simulink model "Quadcopter_sim1NEW"  (R2021a)
settings: Solver=VariableStepAuto  StartTime=0.0  StopTime=t_stop  RelTol=1e-3
values from neighbouring files (symbols this model uses):
  b = 0.001    [Exercise2.m]    (also in Exercise2_3.m)
  Dx = 0.01    [Exercise2.m]    (also in Exercise2_3.m)
  Dy = 0.01    [Exercise2.m]    (also in Exercise2_3.m)
  Dz = 0.01    [Exercise2.m]    (also in Exercise2_3.m)
  g = 9.81    [Exercise2.m]    (also in Exercise2_3.m)
  Ixx = 3e-06    [Exercise2.m]    (also in Exercise2_3.m)
  Iyy = 3e-06    [Exercise2.m]    (also in Exercise2_3.m)
  Izz = 1e-05    [Exercise2.m]    (also in Exercise2_3.m)
  k = 0.01    [Exercise2.m]    (also in Exercise2_3.m)
  L = 0.225    [Exercise2.m]    (also in Exercise2_3.m)
  m = 0.5    [Exercise2.m]    (also in Exercise2_3.m)
  phiSP = phiDegree*pi/180    (= 0)    [Exercise2.m]
  psiSP = psiDegree*pi/180    (= 0)    [Exercise2.m]
  thetaSP = thetaDegree*pi/180    (= 0)    [Exercise2.m]
  zSP = 10    [Exercise2.m]
libraries: pid_lib x4, vrlib x1
settings Model: Creator=emilm  LastModifiedBy=emilm

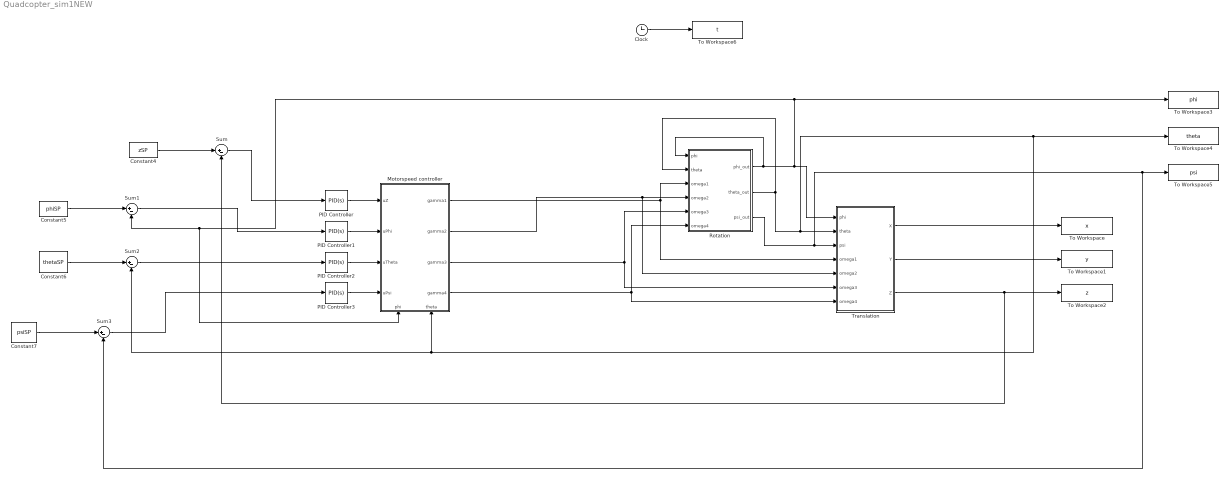
== system Quadcopter_sim1NEW ==
  Clock : Clock
  Constant4 : Constant  Value=zSP
  Constant5 : Constant  Value=phiSP
  Constant6 : Constant  Value=thetaSP
  Constant7 : Constant  Value=psiSP
  Motorspeed controller : Subsystem
      settings: PortSchema="{\"entries\":[{\"content\":{\"sides\":[{\"content\":{\"connectorIds\":[\"In1\",\"In2\",\"In3\",\"In4\"]},\"type\":\"ConnectorPlacement.EquallySpacedRectSide\",\"uuid\":\"02bb1367-ab6e-4bd8-8433-2a069659d175\"},{\"content\":{\"connectorIds\":[\"Out1\",\"Out2\",\"Out3\",\"Out4\"],\"side\":\"RIGHT\"},\"type\":\"ConnectorPlacement.EquallySpacedRectSide\",\"uuid\":\"a63fe295-d221-4681-8f7c-a69bc5358675\"},{\"content\":{\"connectorIds\":[],\"side\":\"TOP\"},\"type\":\"ConnectorPlacement.EquallySpacedRectSide\",\"uuid\":\"253ed6a3-3e04-4ad6-995f-50a6275cee5f\"},{\"content\":{\"connectorIds\":[\"In5\",\"In6\"],\"side\":\"BOTTOM\"},\"type\":\"ConnectorPlacement.EquallySpacedRectSide\",\"uuid\":\"f5e775ff-abe8-4d7a-a704-f626c46163f8\"}]},\"type\":\"ConnectorPlacement.EquallySpacedConnector\",\"uuid\":\"7d3e2221-d52d-4562-8edc-19cce75af537\"}],\"packageUris\":[\"http://schema.mathworks.com/mf0/Connector/R2020b\"],\"version\":\"1.0\"}"
  PID Controller : pid_lib/PID Controller  Controller=PID  Form=Parallel  TimeDomain=Continuous-time  UseExternalTs=off  SampleTime=-1  IntegratorMethod=Forward Euler  FilterMethod=Forward Euler  ControllerParametersSource=internal  P=4.3  I=4.5  D=2  UseFilter=on  N=100  TunerSelectOption=Transfer Function Based (PID Tuner App)  InitialConditionSource=internal  InitialConditionForIntegrator=0  InitialConditionForFilter=0  DifferentiatorICPrevScaledInput=0  ExternalReset=none  TrackingMode=off  Kt=1  LimitOutput=off  SatLimitsSource=internal  UpperSaturationLimit=inf  LowerSaturationLimit=-inf  LinearizeAsGain=on  AntiWindupMode=none  Kb=1  POutMin=[]  POutMax=[]  IOutMin=[]  IOutMax=[]  DOutMin=[]  DOutMax=[]  NOutMin=[]  NOutMax=[]  SumOutMin=[]  SumOutMax=[]  SaturationOutMin=[]  SaturationOutMax=[]  PParamMin=[]  PParamMax=[]  IParamMin=[]  IParamMax=[]  DParamMin=[]  DParamMax=[]  NParamMin=[]  NParamMax=[]  KbParamMin=[]  KbParamMax=[]  KtParamMin=[]  KtParamMax=[]  KbOutMin=[]  KbOutMax=[]  KtOutMin=[]  KtOutMax=[]  IntegratorOutMin=[]  IntegratorOutMax=[]  FilterOutMin=[]  FilterOutMax=[]  SumI1OutMin=[]  SumI1OutMax=[]  SumI2OutMin=[]  SumI2OutMax=[]  SumI3OutMin=[]  SumI3OutMax=[]  SumI4OutMin=[]  SumI4OutMax=[]  SumDOutMin=[]  SumDOutMax=[]  DifferentiatorOutMin=[]  DifferentiatorOutMax=[]  FilterDiffOutCoefMin=[]  FilterDiffOutCoefMax=[]  ReciprocalOutMin=[]  ReciprocalOutMax=[]  SumDenOutMin=[]  SumDenOutMax=[]  SumNumOutMin=[]  SumNumOutMax=[]  DivideOutMin=[]  DivideOutMax=[]  UdiffTsProdOutMin=[]  UdiffTsProdOutMax=[]  NTsProdOutMin=[]  NTsProdOutMax=[]  UintegralTsProdOutMin=[]  UintegralTsProdOutMax=[]  UngainTsProdOutMin=[]  UngainTsProdOutMax=[]  IntegratorContinuousStateAttributes=''  IntegratorStateMustResolveToSignalObject=off  IntegratorRTWStateStorageClass=Auto  FilterContinuousStateAttributes=''  FilterStateMustResolveToSignalObject=off  FilterRTWStateStorageClass=Auto  ParallelPVariant=InternalParameters  IdealPVariant=Disabled  IVariant=InternalParameters  DVariant=InternalParameters  IntegratorVariant=Continuous  SatVariant=Disabled  AWVariant=Passthrough  PCopyVariant=Disabled  TRVariant=Disabled  FdbkBlocksVariant=Forward  IdealPFdbkVariant=Disabled  SatFdbkVariant=Disabled  DerivativeFilterVariant=ContFilter  NVariant=InternalParameters  NCopyVariant=Disabled  FilterICVariant=InternalICsFilter  IntegratorICVariant=InternalICs  ExternalResetVariant=Disabled  TRSumVariant=Passthrough  SumFdbkVariant=Disabled  SumVariant=Sum_PID  TsampFilterVariant=InternalTs  TsampNgainVariant=Passthrough  TsampIntegralVariant=Passthrough  ExternalSaturationOutDataTypeStr=Inherit: Same as second input
  PID Controller1 : pid_lib/PID Controller  Controller=PID  Form=Parallel  TimeDomain=Continuous-time  UseExternalTs=off  SampleTime=-1  IntegratorMethod=Forward Euler  FilterMethod=Forward Euler  ControllerParametersSource=internal  P=0.006  I=0.000009  D=0.013  UseFilter=on  N=100  TunerSelectOption=Transfer Function Based (PID Tuner App)  InitialConditionSource=internal  InitialConditionForIntegrator=0  InitialConditionForFilter=0  DifferentiatorICPrevScaledInput=0  ExternalReset=none  TrackingMode=off  Kt=1  LimitOutput=off  SatLimitsSource=internal  UpperSaturationLimit=inf  LowerSaturationLimit=-inf  LinearizeAsGain=on  AntiWindupMode=none  Kb=1  POutMin=[]  POutMax=[]  IOutMin=[]  IOutMax=[]  DOutMin=[]  DOutMax=[]  NOutMin=[]  NOutMax=[]  SumOutMin=[]  SumOutMax=[]  SaturationOutMin=[]  SaturationOutMax=[]  PParamMin=[]  PParamMax=[]  IParamMin=[]  IParamMax=[]  DParamMin=[]  DParamMax=[]  NParamMin=[]  NParamMax=[]  KbParamMin=[]  KbParamMax=[]  KtParamMin=[]  KtParamMax=[]  KbOutMin=[]  KbOutMax=[]  KtOutMin=[]  KtOutMax=[]  IntegratorOutMin=[]  IntegratorOutMax=[]  FilterOutMin=[]  FilterOutMax=[]  SumI1OutMin=[]  SumI1OutMax=[]  SumI2OutMin=[]  SumI2OutMax=[]  SumI3OutMin=[]  SumI3OutMax=[]  SumI4OutMin=[]  SumI4OutMax=[]  SumDOutMin=[]  SumDOutMax=[]  DifferentiatorOutMin=[]  DifferentiatorOutMax=[]  FilterDiffOutCoefMin=[]  FilterDiffOutCoefMax=[]  ReciprocalOutMin=[]  ReciprocalOutMax=[]  SumDenOutMin=[]  SumDenOutMax=[]  SumNumOutMin=[]  SumNumOutMax=[]  DivideOutMin=[]  DivideOutMax=[]  UdiffTsProdOutMin=[]  UdiffTsProdOutMax=[]  NTsProdOutMin=[]  NTsProdOutMax=[]  UintegralTsProdOutMin=[]  UintegralTsProdOutMax=[]  UngainTsProdOutMin=[]  UngainTsProdOutMax=[]  IntegratorContinuousStateAttributes=''  IntegratorStateMustResolveToSignalObject=off  IntegratorRTWStateStorageClass=Auto  FilterContinuousStateAttributes=''  FilterStateMustResolveToSignalObject=off  FilterRTWStateStorageClass=Auto  ParallelPVariant=InternalParameters  IdealPVariant=Disabled  IVariant=InternalParameters  DVariant=InternalParameters  IntegratorVariant=Continuous  SatVariant=Disabled  AWVariant=Passthrough  PCopyVariant=Disabled  TRVariant=Disabled  FdbkBlocksVariant=Forward  IdealPFdbkVariant=Disabled  SatFdbkVariant=Disabled  DerivativeFilterVariant=ContFilter  NVariant=InternalParameters  NCopyVariant=Disabled  FilterICVariant=InternalICsFilter  IntegratorICVariant=InternalICs  ExternalResetVariant=Disabled  TRSumVariant=Passthrough  SumFdbkVariant=Disabled  SumVariant=Sum_PID  TsampFilterVariant=InternalTs  TsampNgainVariant=Passthrough  TsampIntegralVariant=Passthrough  ExternalSaturationOutDataTypeStr=Inherit: Same as second input
  PID Controller2 : pid_lib/PID Controller  Controller=PID  Form=Parallel  TimeDomain=Continuous-time  UseExternalTs=off  SampleTime=-1  IntegratorMethod=Forward Euler  FilterMethod=Forward Euler  ControllerParametersSource=internal  P=0.006  I=0.000009  D=0.013  UseFilter=on  N=100  TunerSelectOption=Transfer Function Based (PID Tuner App)  InitialConditionSource=internal  InitialConditionForIntegrator=0  InitialConditionForFilter=0  DifferentiatorICPrevScaledInput=0  ExternalReset=none  TrackingMode=off  Kt=1  LimitOutput=off  SatLimitsSource=internal  UpperSaturationLimit=inf  LowerSaturationLimit=-inf  LinearizeAsGain=on  AntiWindupMode=none  Kb=1  POutMin=[]  POutMax=[]  IOutMin=[]  IOutMax=[]  DOutMin=[]  DOutMax=[]  NOutMin=[]  NOutMax=[]  SumOutMin=[]  SumOutMax=[]  SaturationOutMin=[]  SaturationOutMax=[]  PParamMin=[]  PParamMax=[]  IParamMin=[]  IParamMax=[]  DParamMin=[]  DParamMax=[]  NParamMin=[]  NParamMax=[]  KbParamMin=[]  KbParamMax=[]  KtParamMin=[]  KtParamMax=[]  KbOutMin=[]  KbOutMax=[]  KtOutMin=[]  KtOutMax=[]  IntegratorOutMin=[]  IntegratorOutMax=[]  FilterOutMin=[]  FilterOutMax=[]  SumI1OutMin=[]  SumI1OutMax=[]  SumI2OutMin=[]  SumI2OutMax=[]  SumI3OutMin=[]  SumI3OutMax=[]  SumI4OutMin=[]  SumI4OutMax=[]  SumDOutMin=[]  SumDOutMax=[]  DifferentiatorOutMin=[]  DifferentiatorOutMax=[]  FilterDiffOutCoefMin=[]  FilterDiffOutCoefMax=[]  ReciprocalOutMin=[]  ReciprocalOutMax=[]  SumDenOutMin=[]  SumDenOutMax=[]  SumNumOutMin=[]  SumNumOutMax=[]  DivideOutMin=[]  DivideOutMax=[]  UdiffTsProdOutMin=[]  UdiffTsProdOutMax=[]  NTsProdOutMin=[]  NTsProdOutMax=[]  UintegralTsProdOutMin=[]  UintegralTsProdOutMax=[]  UngainTsProdOutMin=[]  UngainTsProdOutMax=[]  IntegratorContinuousStateAttributes=''  IntegratorStateMustResolveToSignalObject=off  IntegratorRTWStateStorageClass=Auto  FilterContinuousStateAttributes=''  FilterStateMustResolveToSignalObject=off  FilterRTWStateStorageClass=Auto  ParallelPVariant=InternalParameters  IdealPVariant=Disabled  IVariant=InternalParameters  DVariant=InternalParameters  IntegratorVariant=Continuous  SatVariant=Disabled  AWVariant=Passthrough  PCopyVariant=Disabled  TRVariant=Disabled  FdbkBlocksVariant=Forward  IdealPFdbkVariant=Disabled  SatFdbkVariant=Disabled  DerivativeFilterVariant=ContFilter  NVariant=InternalParameters  NCopyVariant=Disabled  FilterICVariant=InternalICsFilter  IntegratorICVariant=InternalICs  ExternalResetVariant=Disabled  TRSumVariant=Passthrough  SumFdbkVariant=Disabled  SumVariant=Sum_PID  TsampFilterVariant=InternalTs  TsampNgainVariant=Passthrough  TsampIntegralVariant=Passthrough  ExternalSaturationOutDataTypeStr=Inherit: Same as second input
  PID Controller3 : pid_lib/PID Controller  Controller=PID  Form=Parallel  TimeDomain=Continuous-time  UseExternalTs=off  SampleTime=-1  IntegratorMethod=Forward Euler  FilterMethod=Forward Euler  ControllerParametersSource=internal  P=0.01  I=0.0002  D=0.03  UseFilter=on  N=100  TunerSelectOption=Transfer Function Based (PID Tuner App)  InitialConditionSource=internal  InitialConditionForIntegrator=0  InitialConditionForFilter=0  DifferentiatorICPrevScaledInput=0  ExternalReset=none  TrackingMode=off  Kt=1  LimitOutput=off  SatLimitsSource=internal  UpperSaturationLimit=inf  LowerSaturationLimit=-inf  LinearizeAsGain=on  AntiWindupMode=none  Kb=1  POutMin=[]  POutMax=[]  IOutMin=[]  IOutMax=[]  DOutMin=[]  DOutMax=[]  NOutMin=[]  NOutMax=[]  SumOutMin=[]  SumOutMax=[]  SaturationOutMin=[]  SaturationOutMax=[]  PParamMin=[]  PParamMax=[]  IParamMin=[]  IParamMax=[]  DParamMin=[]  DParamMax=[]  NParamMin=[]  NParamMax=[]  KbParamMin=[]  KbParamMax=[]  KtParamMin=[]  KtParamMax=[]  KbOutMin=[]  KbOutMax=[]  KtOutMin=[]  KtOutMax=[]  IntegratorOutMin=[]  IntegratorOutMax=[]  FilterOutMin=[]  FilterOutMax=[]  SumI1OutMin=[]  SumI1OutMax=[]  SumI2OutMin=[]  SumI2OutMax=[]  SumI3OutMin=[]  SumI3OutMax=[]  SumI4OutMin=[]  SumI4OutMax=[]  SumDOutMin=[]  SumDOutMax=[]  DifferentiatorOutMin=[]  DifferentiatorOutMax=[]  FilterDiffOutCoefMin=[]  FilterDiffOutCoefMax=[]  ReciprocalOutMin=[]  ReciprocalOutMax=[]  SumDenOutMin=[]  SumDenOutMax=[]  SumNumOutMin=[]  SumNumOutMax=[]  DivideOutMin=[]  DivideOutMax=[]  UdiffTsProdOutMin=[]  UdiffTsProdOutMax=[]  NTsProdOutMin=[]  NTsProdOutMax=[]  UintegralTsProdOutMin=[]  UintegralTsProdOutMax=[]  UngainTsProdOutMin=[]  UngainTsProdOutMax=[]  IntegratorContinuousStateAttributes=''  IntegratorStateMustResolveToSignalObject=off  IntegratorRTWStateStorageClass=Auto  FilterContinuousStateAttributes=''  FilterStateMustResolveToSignalObject=off  FilterRTWStateStorageClass=Auto  ParallelPVariant=InternalParameters  IdealPVariant=Disabled  IVariant=InternalParameters  DVariant=InternalParameters  IntegratorVariant=Continuous  SatVariant=Disabled  AWVariant=Passthrough  PCopyVariant=Disabled  TRVariant=Disabled  FdbkBlocksVariant=Forward  IdealPFdbkVariant=Disabled  SatFdbkVariant=Disabled  DerivativeFilterVariant=ContFilter  NVariant=InternalParameters  NCopyVariant=Disabled  FilterICVariant=InternalICsFilter  IntegratorICVariant=InternalICs  ExternalResetVariant=Disabled  TRSumVariant=Passthrough  SumFdbkVariant=Disabled  SumVariant=Sum_PID  TsampFilterVariant=InternalTs  TsampNgainVariant=Passthrough  TsampIntegralVariant=Passthrough  ExternalSaturationOutDataTypeStr=Inherit: Same as second input
  Rotation : Subsystem
  Sum{,1..3} (4 alike) : Sum  Inputs=|+-
  To Workspace : ToWorkspace  VariableName=x  SampleTime=-1
  To Workspace1 : ToWorkspace  VariableName=y  SampleTime=-1
  To Workspace2 : ToWorkspace  VariableName=z  SampleTime=-1
  To Workspace3 : ToWorkspace  VariableName=phi  SampleTime=-1
  To Workspace4 : ToWorkspace  VariableName=theta  SampleTime=-1
  To Workspace5 : ToWorkspace  VariableName=psi  SampleTime=-1
  To Workspace6 : ToWorkspace  VariableName=t  SampleTime=-1
  Translation : Subsystem
  wires:
  Rotation/1(phi_out) -> Rotation/1(phi), To Workspace3/1, Sum1/2, Motorspeed controller/5(phi), Translation/1(phi)
  Rotation/2(theta_out) -> To Workspace4/1, Motorspeed controller/6(theta), Sum2/2, Translation/2(theta), Rotation/2(theta)
  Rotation/3(psi_out) -> To Workspace5/1, Sum3/2, Translation/3(psi)
  Motorspeed controller/1(gamma1) -> Rotation/3(omega1), Translation/4(omega1)
  Motorspeed controller/2(gamma2) -> Translation/5(omega2), Rotation/4(omega2)
  Motorspeed controller/3(gamma3) -> Translation/6(omega3), Rotation/5(omega3)
  Motorspeed controller/4(gamma4) -> Translation/7(omega4), Rotation/6(omega4)
  Translation/1(X) -> To Workspace/1
  Translation/2(Y) -> To Workspace1/1
  Translation/3(Z) -> Sum/2, To Workspace2/1
  Clock/1 -> To Workspace6/1
  PID Controller/1 -> Motorspeed controller/1(uZ)
  PID Controller1/1 -> Motorspeed controller/2(uPhi)
  PID Controller2/1 -> Motorspeed controller/3(uTheta)
  PID Controller3/1 -> Motorspeed controller/4(uPsi)
  Constant4/1 -> Sum/1
  Constant5/1 -> Sum1/1
  Constant6/1 -> Sum2/1
  Constant7/1 -> Sum3/1
  Sum/1 -> PID Controller/1
  Sum1/1 -> PID Controller1/1
  Sum2/1 -> PID Controller2/1
  Sum3/1 -> PID Controller3/1

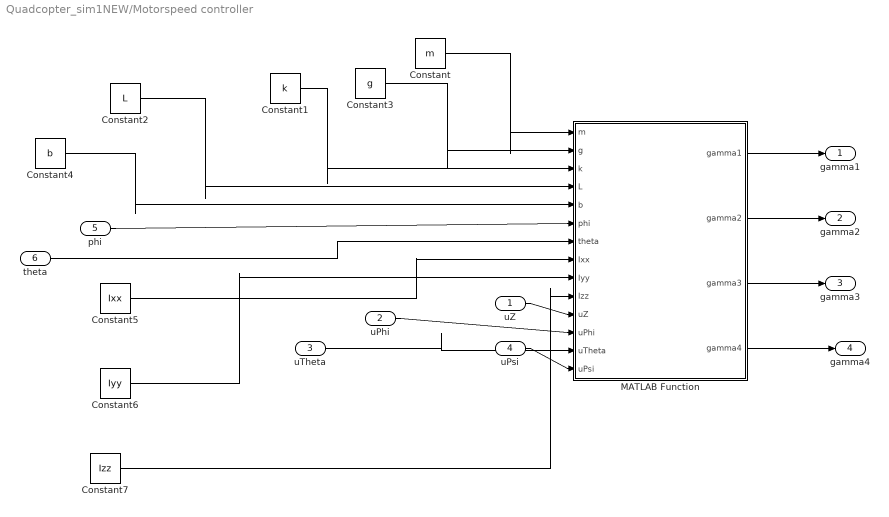
== system Quadcopter_sim1NEW/Motorspeed controller ==
  uZ : Inport
  uPhi : Inport  Port=2
  uTheta : Inport  Port=3
  uPsi : Inport  Port=4
  phi : Inport  Port=5
  theta : Inport  Port=6
  Constant : Constant  Value=m
  Constant1 : Constant  Value=k
  Constant2 : Constant  Value=L
  Constant3 : Constant  Value=g
  Constant4 : Constant  Value=b
  Constant5 : Constant  Value=Ixx
  Constant6 : Constant  Value=Iyy
  Constant7 : Constant  Value=Izz
  MATLAB Function : MATLAB Function  TreatAsAtomicUnit=on
  gamma1 : Outport
  gamma2 : Outport  Port=2
  gamma3 : Outport  Port=3
  gamma4 : Outport  Port=4
  wires:
  MATLAB Function/1(gamma1) -> gamma1/1
  MATLAB Function/2(gamma2) -> gamma2/1
  MATLAB Function/3(gamma3) -> gamma3/1
  MATLAB Function/4(gamma4) -> gamma4/1
  uZ/1 -> MATLAB Function/11(uZ)
  uPsi/1 -> MATLAB Function/14(uPsi)
  uPhi/1 -> MATLAB Function/12(uPhi)
  uTheta/1 -> MATLAB Function/13(uTheta)
  phi/1 -> MATLAB Function/6(phi)
  theta/1 -> MATLAB Function/7(theta)
  Constant/1 -> MATLAB Function/1(m)
  Constant3/1 -> MATLAB Function/2(g)
  Constant1/1 -> MATLAB Function/3(k)
  Constant2/1 -> MATLAB Function/4(L)
  Constant4/1 -> MATLAB Function/5(b)
  Constant5/1 -> MATLAB Function/8(Ixx)
  Constant6/1 -> MATLAB Function/9(Iyy)
  Constant7/1 -> MATLAB Function/10(Izz)

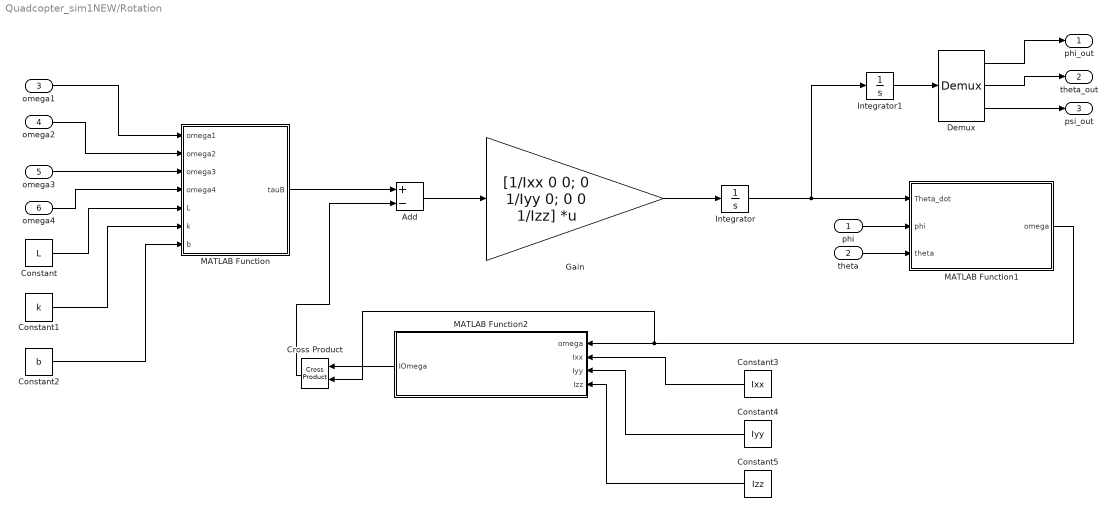
== system Quadcopter_sim1NEW/Rotation ==
  phi : Inport
  theta : Inport  Port=2
  omega1 : Inport  Port=3
  omega2 : Inport  Port=4
  omega3 : Inport  Port=5
  omega4 : Inport  Port=6
  Add : Sum  Inputs=+-
  Constant : Constant  Value=L
  Constant1 : Constant  Value=k
  Constant2 : Constant  Value=b
  Constant3 : Constant  Value=Ixx
  Constant4 : Constant  Value=Iyy
  Constant5 : Constant  Value=Izz
  Cross Product : vrlib/Utilities/Cross Product
  Demux : Demux  Outputs=3
  Gain : Gain  Gain=[1/Ixx 0 0; 0 1/Iyy 0; 0 0 1/Izz]  Multiplication=Matrix(K*u)
  Integrator : Integrator
  Integrator1 : Integrator
  MATLAB Function : MATLAB Function  TreatAsAtomicUnit=on
  MATLAB Function1 : MATLAB Function  TreatAsAtomicUnit=on
  MATLAB Function2 : MATLAB Function  TreatAsAtomicUnit=on
  phi_out : Outport
  theta_out : Outport  Port=2
  psi_out : Outport  Port=3
  wires:
  omega1/1 -> MATLAB Function/1(omega1)
  omega2/1 -> MATLAB Function/2(omega2)
  omega3/1 -> MATLAB Function/3(omega3)
  omega4/1 -> MATLAB Function/4(omega4)
  Constant/1 -> MATLAB Function/5(L)
  Constant1/1 -> MATLAB Function/6(k)
  Constant2/1 -> MATLAB Function/7(b)
  MATLAB Function/1(tauB) -> Add/1
  Add/1 -> Gain/1
  Gain/1 -> Integrator/1
  Integrator/1 -> Integrator1/1, MATLAB Function1/1(Theta_dot)
  phi/1 -> MATLAB Function1/2(phi)
  theta/1 -> MATLAB Function1/3(theta)
  MATLAB Function1/1(omega) -> Cross Product/2, MATLAB Function2/1(omega)
  Integrator1/1 -> Demux/1
  Demux/1 -> phi_out/1
  Demux/2 -> theta_out/1
  Demux/3 -> psi_out/1
  Constant3/1 -> MATLAB Function2/2(Ixx)
  Constant4/1 -> MATLAB Function2/3(Iyy)
  Constant5/1 -> MATLAB Function2/4(Izz)
  MATLAB Function2/1(IOmega) -> Cross Product/1
  Cross Product/1 -> Add/2

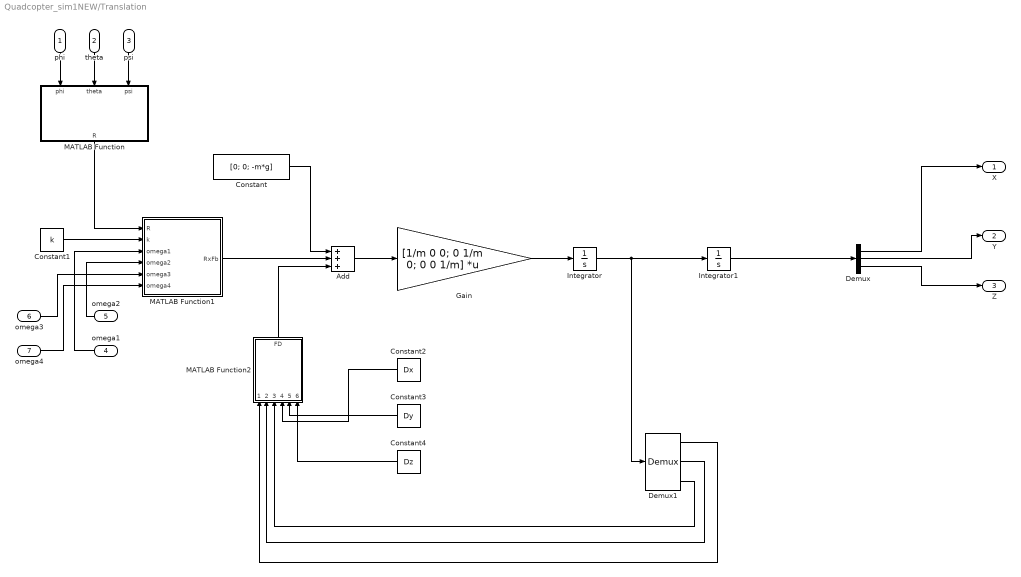
== system Quadcopter_sim1NEW/Translation ==
  phi : Inport
  theta : Inport  Port=2
  psi : Inport  Port=3
  omega1 : Inport  Port=4
  omega2 : Inport  Port=5
  omega3 : Inport  Port=6
  omega4 : Inport  Port=7
  Add : Sum  Inputs=+++
  Constant : Constant  Value=[0; 0; -m*g]
  Constant1 : Constant  Value=k
  Constant2 : Constant  Value=Dx
  Constant3 : Constant  Value=Dy
  Constant4 : Constant  Value=Dz
  Demux : Demux  Outputs=3
  Demux1 : Demux  Outputs=3
  Gain : Gain  Gain=[1/m 0 0; 0 1/m 0; 0 0 1/m]  Multiplication=Matrix(K*u)
  Integrator : Integrator
  Integrator1 : Integrator
  MATLAB Function : MATLAB Function  TreatAsAtomicUnit=on
  MATLAB Function1 : MATLAB Function  TreatAsAtomicUnit=on
  MATLAB Function2 : MATLAB Function  TreatAsAtomicUnit=on
  X : Outport
  Y : Outport  Port=2
  Z : Outport  Port=3
  wires:
  Gain/1 -> Integrator/1
  theta/1 -> MATLAB Function/2(theta)
  psi/1 -> MATLAB Function/3(psi)
  phi/1 -> MATLAB Function/1(phi)
  Add/1 -> Gain/1
  Constant/1 -> Add/1
  MATLAB Function1/1(RxFb) -> Add/2
  MATLAB Function/1(R) -> MATLAB Function1/1(R)
  Constant1/1 -> MATLAB Function1/2(k)
  omega2/1 -> MATLAB Function1/4(omega2)
  omega1/1 -> MATLAB Function1/3(omega1)
  omega3/1 -> MATLAB Function1/5(omega3)
  omega4/1 -> MATLAB Function1/6(omega4)
  Integrator/1 -> Demux1/1, Integrator1/1
  Integrator1/1 -> Demux/1
  Demux/1 -> X/1
  Demux/2 -> Y/1
  Demux/3 -> Z/1
  MATLAB Function2/1(FD) -> Add/3
  Constant2/1 -> MATLAB Function2/4(Dx)
  Constant3/1 -> MATLAB Function2/5(Dy)
  Constant4/1 -> MATLAB Function2/6(Dz)
  Demux1/1 -> MATLAB Function2/1(x_dot)
  Demux1/2 -> MATLAB Function2/2(y_dot)
  Demux1/3 -> MATLAB Function2/3(z_dot)

== matlab function Quadcopter_sim1NEW/Translation/MATLAB Function1 ==
  data: R input; RxFb output; k input; omega1 input; omega2 input; omega3 input; omega4 input
function RxFb = RxFb(R, k, omega1, omega2, omega3, omega4)

RxFb = R*[0; 0; k*(omega1+omega2+omega3+omega4)];

== matlab function Quadcopter_sim1NEW/Translation/MATLAB Function ==
  data: phi input; R output; theta input; psi input
function R = R(phi, theta, psi)

c1 = cos(phi);
c2 = cos(theta);
c3 = cos(psi);

s1 = sin(phi);
s2 = sin(theta);
s3 = sin(psi);


R = [c3*c2 c3*s2*s1-s3*c1 c3*s2*c1+s3*s1;
     s3*c2 s3*s2*s1+c3*c1 s3*s2*c1-c3*s1
     -s2         c2*s1        c2*c1];

== matlab function Quadcopter_sim1NEW/Translation/MATLAB Function2 ==
  data: x_dot input; y_dot input; z_dot input; FD output; Dx input; Dy input; Dz input
function FD = FD(x_dot, y_dot, z_dot, Dx, Dy, Dz)

D = [Dx 0 0; 0 Dy 0; 0 0 Dz];

FD = D*[x_dot; y_dot; z_dot];

== matlab function Quadcopter_sim1NEW/Rotation/MATLAB Function ==
  data: omega1 input; tauB output; omega2 input; omega3 input; omega4 input; L input; k input; b input
function tauB = tauB(omega1, omega2, omega3, omega4, L, k, b)

tauB = [L*k*(omega1-omega3);
        L*k*(omega2-omega4);
        b*(omega1-omega2+omega3-omega4)];

== matlab function Quadcopter_sim1NEW/Rotation/MATLAB Function1 ==
  data: Theta_dot input; omega output; phi input; theta input
function omega = omega(Theta_dot, phi, theta)

R = [1 0 -sin(theta);
     0 cos(phi) cos(theta)*sin(phi);
     0 -sin(phi) cos(theta)*cos(phi)];
 
 omega = R*Theta_dot;

== matlab function Quadcopter_sim1NEW/Rotation/MATLAB Function2 ==
  data: omega input; IOmega output; Ixx input; Iyy input; Izz input
function IOmega = Iomega(omega, Ixx, Iyy, Izz)



IOmega = [Ixx 0 0; 0 Iyy 0; 0 0 Izz]*omega;

== matlab function Quadcopter_sim1NEW/Motorspeed controller/MATLAB Function ==
  data: m input; gamma1 output; g input; k input; L input; b input; phi input; theta input; Ixx input; Iyy input; Izz input; uZ input; uPhi input; uTheta input; uPsi input; gamma2 output; gamma3 output; gamma4 output
function [gamma1,gamma2, gamma3, gamma4]= MotorSpeed(m, g, k, L, b, phi, theta, Ixx, Iyy, Izz, uZ, uPhi, uTheta, uPsi)

gamma1 = ((m*g+uZ*m)/(k*4*cos(theta)*cos(phi)))-((2*b*uPhi*Ixx+uPsi*Izz*k*L)/(4*b*k*L));

gamma2 = ((m*g+uZ*m)/(k*4*cos(theta)*cos(phi)))-((2*b*uTheta*Iyy-uPsi*Izz*k*L)/(4*b*k*L));

gamma3 = ((m*g+uZ*m)/(k*4*cos(theta)*cos(phi)))-((-2*b*uPhi*Ixx+uPsi*Izz*k*L)/(4*b*k*L));

gamma4 = ((m*g+uZ*m)/(k*4*cos(theta)*cos(phi)))-((-2*b*uTheta*Iyy-uPsi*Izz*k*L)/(4*b*k*L));
